simulink model "lcl_fo"  (R2015a)
settings: Solver=ode45  StartTime=0.0  StopTime=.04  MaxStep=Ts/1000  RelTol=1e-3
values from neighbouring files (symbols this model uses):
  A = [a11, a12, a13 ... (first row only)    [Sim_lcl_fo.m]    (also in Sim_lcl_ro.m)
  Bc = [bc1; bc2; bc3]    [Sim_lcl_fo.m]    (also in Sim_lcl_ro.m)
  K = Ka(1:4)    [Sim_lcl_fo.m]    (also in Sim_lcl_ro.m)
  ki = -Ka(5)    [Sim_lcl_fo.m]    (also in Sim_lcl_ro.m)
  Ko = acker(A',Cc',po).'    [Sim_lcl_fo.m]
  kt = ki/(1 - beta)    [Sim_lcl_fo.m]    (also in Sim_lcl_ro.m)
  sigmaNoise = 0*.1    (= 0)    [Sim_lcl_fo.m]    (also in Sim_lcl_ro.m)
  TNoise = Ts    (= 0.0002)    [Sim_lcl_fo.m]    (also in Sim_lcl_ro.m = 0.0001)
  Ts = 200e-6    (= 0.0002)    [Sim_lcl_fo.m]    (also in Sim_lcl_ro.m = 0.0001)
  Tsw = Ts    (= 0.0002)    [Sim_lcl_fo.m]    (also in Sim_lcl_ro.m = 0.0001)
  Udc = 350    [Sim_lcl_fo.m]    (also in Sim_lcl_ro.m)
  ug0 = ug0Act    (= 300)    [Sim_lcl_fo.m]    (also in Sim_lcl_ro.m)
  ug0Act = 300    [Sim_lcl_fo.m]    (also in Sim_lcl_ro.m)
  ui0 = ug0 + K*[xEst0; ug0]    [Sim_lcl_fo.m]    (also in Sim_lcl_ro.m = ug0 + K*xdEst0)
  uMax = Udc    (= 350)    [Sim_lcl_fo.m]    (also in Sim_lcl_ro.m)
  xEst0 = (eye(3) - A + Ko*Cc)\Bc*ug0    [Sim_lcl_fo.m]
undefined symbols (not defined in the file): CfAct, LfcAct, LfgAct
libraries: simulink x2
settings Model: Creator=mhink  LastModifiedBy=mhinkkan
settings DataIOCC: SaveFormat=Dataset
settings HardwareCC: ProdBitPerPointer=64  ProdLargestAtomicFloat=Float  ProdIntDivRoundTo=Zero  ProdEndianess=LittleEndian  ProdHWDeviceType=Specified
settings GRTTargetCC: GeneratePreprocessorConditionals=Use local settings

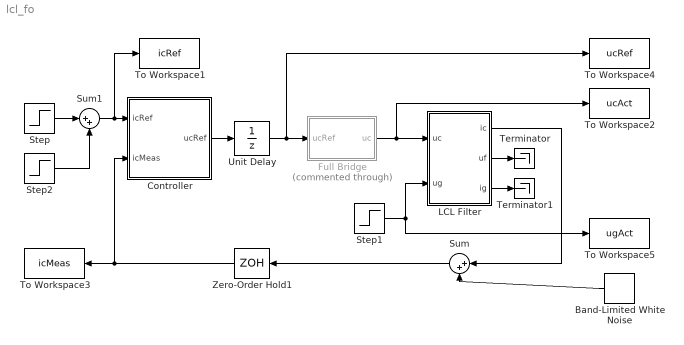
== system lcl_fo ==
  Band-Limited White Noise : simulink/Sources/Band-Limited White Noise  Cov=[sigmaNoise^2*TNoise]  Ts=TNoise  seed=[23341]
  Controller : Subsystem
  Full Bridge : Subsystem  Commented=through
  LCL Filter : Subsystem  mask{Lfc=LfcAct, Cf=CfAct, Lfg=LfgAct, ug0=ug0Act}
      mask prompts: Lfc "Converter-side inductance Lfc (H)"; Cf "Capacitance Cf (F)"; Lfg "Grid-side inductance Lfg (H)"; ug0 "Initial value ug0 (V)"
  Step : Step  Time=.002  After=10  SampleTime=Ts
  Step1 : Step  Time=.01  Before=ug0Act  After=200  SampleTime=0
  Step2 : Step  Time=.02  After=10  SampleTime=Ts
  Sum : Sum  Inputs=|++
  Sum1 : Sum  Inputs=|++
  Terminator : Terminator
  Terminator1 : Terminator
  To Workspace1 : ToWorkspace  VariableName=icRef  SaveFormat=Timeseries  SampleTime=-1
  To Workspace2 : ToWorkspace  VariableName=ucAct  SaveFormat=Timeseries  SampleTime=-1
  To Workspace3 : ToWorkspace  VariableName=icMeas  SaveFormat=Timeseries  SampleTime=-1
  To Workspace4 : ToWorkspace  VariableName=ucRef  SaveFormat=Timeseries  SampleTime=-1
  To Workspace5 : ToWorkspace  VariableName=ugAct  SaveFormat=Timeseries  SampleTime=Ts
  Unit Delay : UnitDelay  InitialCondition=ug0  SampleTime=Ts
  Zero-Order Hold1 : ZeroOrderHold  SampleTime=Ts
  wires:
  Controller/1(ucRef) -> Unit Delay/1
  Full Bridge/1(uc) -> LCL Filter/1(uc), To Workspace2/1
  Zero-Order Hold1/1 -> To Workspace3/1, Controller/2(icMeas)
  Step1/1 -> To Workspace5/1, LCL Filter/2(ug)
  Unit Delay/1 -> Full Bridge/1(ucRef), To Workspace4/1
  LCL Filter/1(ic) -> Sum/1
  Sum/1 -> Zero-Order Hold1/1
  Band-Limited White Noise/1 -> Sum/2
  Step/1 -> Sum1/1
  Sum1/1 -> To Workspace1/1, Controller/1(icRef)
  Step2/1 -> Sum1/2
  LCL Filter/2(uf) -> Terminator/1
  LCL Filter/3(ig) -> Terminator1/1

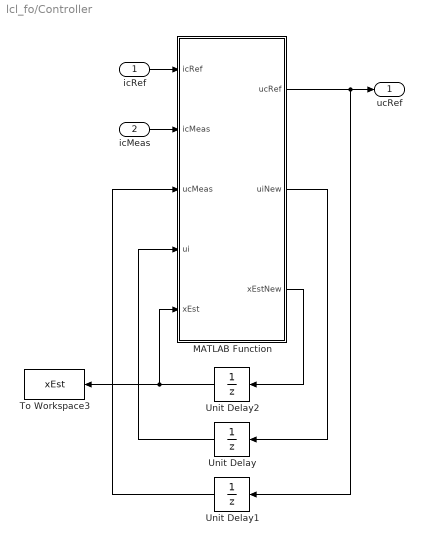
== system lcl_fo/Controller ==
  icRef : Inport
  icMeas : Inport  Port=2
  MATLAB Function : MATLAB Function  TreatAsAtomicUnit=on
      settings: PermitHierarchicalResolution=ParametersOnly
  To Workspace3 : ToWorkspace  VariableName=xEst  SaveFormat=Timeseries  SampleTime=-1
  Unit Delay : UnitDelay  InitialCondition=ui0  SampleTime=Ts
  Unit Delay1 : UnitDelay  InitialCondition=ug0  SampleTime=Ts
  Unit Delay2 : UnitDelay  InitialCondition=xEst0  SampleTime=Ts
  ucRef : Outport
  wires:
  MATLAB Function/2(uiNew) -> Unit Delay/1
  icRef/1 -> MATLAB Function/1(icRef)
  MATLAB Function/1(ucRef) -> ucRef/1, Unit Delay1/1
  Unit Delay/1 -> MATLAB Function/4(ui)
  icMeas/1 -> MATLAB Function/2(icMeas)
  MATLAB Function/3(xEstNew) -> Unit Delay2/1
  Unit Delay2/1 -> MATLAB Function/5(xEst), To Workspace3/1
  Unit Delay1/1 -> MATLAB Function/3(ucMeas)

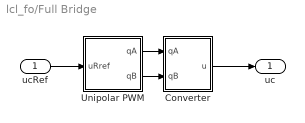
== system lcl_fo/Full Bridge ==
  ucRef : Inport
  Converter : Subsystem
  Unipolar PWM : Subsystem
  uc : Outport
  wires:
  Converter/1(u) -> uc/1
  Unipolar PWM/2(qB) -> Converter/2(qB)
  Unipolar PWM/1(qA) -> Converter/1(qA)
  ucRef/1 -> Unipolar PWM/1(uRref)

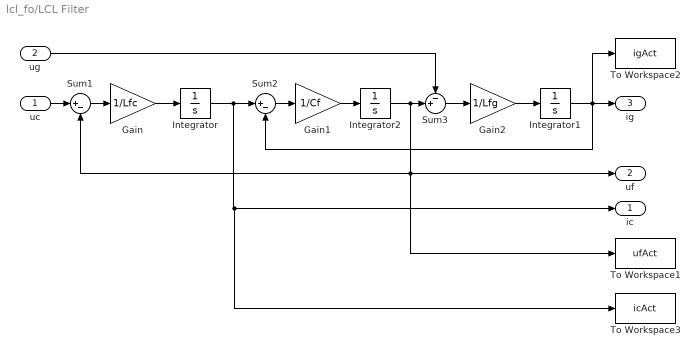
== system lcl_fo/LCL Filter ==
  uc : Inport
  ug : Inport  Port=2
  Gain : Gain  Gain=1/Lfc
  Gain1 : Gain  Gain=1/Cf
  Gain2 : Gain  Gain=1/Lfg
  Integrator : Integrator
  Integrator1 : Integrator
  Integrator2 : Integrator  InitialCondition=ug0
  Sum1 : Sum  Inputs=|+-
  Sum2 : Sum  Inputs=|+-
  Sum3 : Sum  Inputs=-+|
  To Workspace1 : ToWorkspace  VariableName=ufAct  SaveFormat=Timeseries  SampleTime=-1
  To Workspace2 : ToWorkspace  VariableName=igAct  SaveFormat=Timeseries  SampleTime=-1
  To Workspace3 : ToWorkspace  VariableName=icAct  SaveFormat=Timeseries  SampleTime=-1
  ic : Outport
  uf : Outport  Port=2
  ig : Outport  Port=3
  wires:
  uc/1 -> Sum1/1
  Sum1/1 -> Gain/1
  Gain/1 -> Integrator/1
  Integrator/1 -> To Workspace3/1, ic/1, Sum2/1
  Sum2/1 -> Gain1/1
  Gain1/1 -> Integrator2/1
  Sum3/1 -> Gain2/1
  Integrator1/1 -> To Workspace2/1, Sum2/2, ig/1
  Gain2/1 -> Integrator1/1
  Integrator2/1 -> To Workspace1/1, Sum1/2, uf/1, Sum3/2
  ug/1 -> Sum3/1

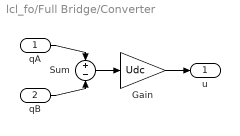
== system lcl_fo/Full Bridge/Converter ==
  qA : Inport
  qB : Inport  Port=2
  Gain : Gain  Gain=Udc
  Sum : Sum  Inputs=+|-
  u : Outport
  wires:
  qA/1 -> Sum/1
  qB/1 -> Sum/2
  Gain/1 -> u/1
  Sum/1 -> Gain/1

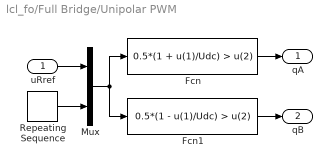
== system lcl_fo/Full Bridge/Unipolar PWM ==
  uRref : Inport
  Fcn : Fcn  Expr=0.5*(1 + u(1)/Udc) > u(2)
  Fcn1 : Fcn  Expr=0.5*(1 - u(1)/Udc) > u(2)
  Mux : Mux  Inputs=2
  Repeating Sequence : simulink/Sources/Repeating Sequence  rep_seq_t=Tsw*[0 0.5 1]  rep_seq_y=[1 0 1]
  qA : Outport
  qB : Outport  Port=2
  wires:
  uRref/1 -> Mux/1
  Mux/1 -> Fcn1/1, Fcn/1
  Repeating Sequence/1 -> Mux/2
  Fcn/1 -> qA/1
  Fcn1/1 -> qB/1

== matlab function lcl_fo/Controller/MATLAB Function ==
  data: icRef input size=1; ucRef output size=1; icMeas input; ucMeas input; ui input size=1; uiNew output size=1; uMax parameter; kt parameter; K parameter; ki parameter; xEst input; xEstNew output; A parameter; Bc parameter; Ko parameter
function [ucRef,uiNew,xEstNew] = fcn(icRef,icMeas, ucMeas,ui,uMax,kt,K, ki, xEst,A, Bc, Ko)

% Calculate the ideal controller output
xd = [xEst; ucMeas];
ucRefIdeal = kt*icRef - K*xd + ui;

% Limit the output
ucRef = ucRefIdeal;
if(ucRef > uMax)
    ucRef = uMax;
elseif(ucRef < -uMax)
    ucRef = -uMax;
end

% Update the integrator state. Last term is the antiwindup.
uiNew = ui + ki*((icRef - icMeas) + (ucRef - ucRefIdeal)/kt);

icEst = xEst(1); 
xEstNew = A*xEst + Bc*ucMeas + Ko*(icMeas - icEst);
